simulink model "pid_line_following"  (R2016b)
settings: Solver=FixedStepAuto  StartTime=0.0  StopTime=10.0  RelTol=1e-3  EnableMultiTasking=on
libraries: legoev3lib x6
settings Model: ExtModeTrigDuration=2  Creator=Nexel  LastModifiedBy=Nexel
settings SolverCC: PositivePriorityOrder=on
settings OptimizationCC: MaxStackSize=64
settings DebuggingCC: ParameterTunabilityLossMsg=error
settings HardwareCC: ProdBitPerPointer=32  ProdBitPerSizeT=32  ProdBitPerPtrDiffT=32  ProdLargestAtomicInteger=Long  ProdWordSize=32  ProdHWDeviceType=ARM Compatible->ARM 9
settings RTWCC: SystemTargetFile=ert.tlc  HardwareBoard=LEGO MINDSTORMS EV3  TLCOptions="-aInlineSetEventsForThisBaseRateFcn=TLC_FALSE -aSuppressMultiTaskScheduler=TLC_FALSE  -aRateBasedStepFcn=0"  TemplateMakefile=ert_default_tmf  Description=Embedded Coder  GenerateReport=on  Toolchain=Sourcery G++ Lite v2009q3  IncludeHyperlinkInReport=on  LaunchReport=on  GenerateTraceInfo=on  GenerateTraceReport=on  GenerateTraceReportSl=on  GenerateTraceReportSf=on  GenerateTraceReportEml=on
settings CodeAppCC: ForceParamTrailComments=on  IgnoreCustomStorageClasses=off  OperatorAnnotations=on  SimulinkDataObjDesc=on  SFDataObjDesc=on  MATLABFcnDesc=on  InsertBlockDesc=on  MATLABSourceComments=on
settings ERTTargetCC: SupportContinuousTime=on  SupportVariableSizeSignals=on

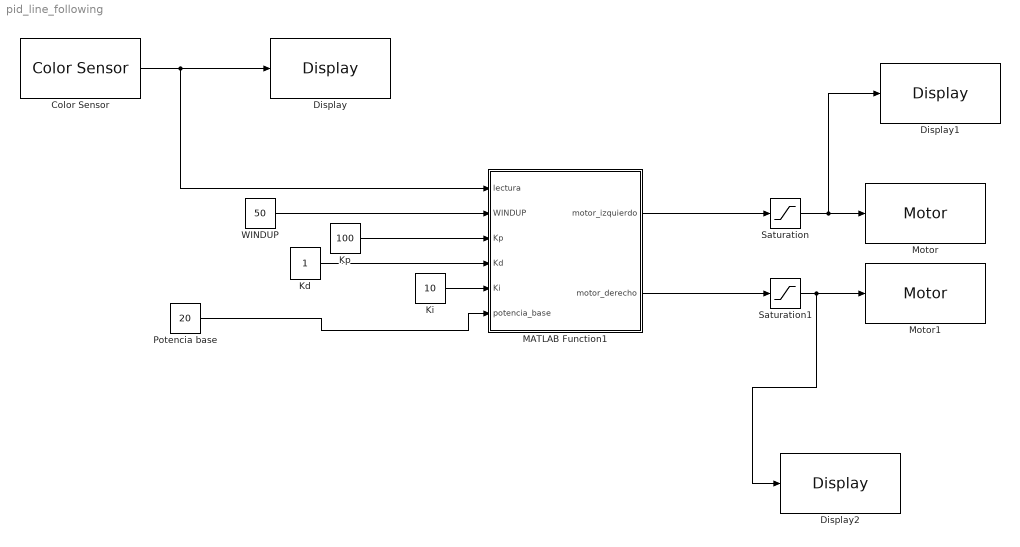
== system pid_line_following ==
  Color Sensor : legoev3lib/Color Sensor  portNumber=1  mode=Reflected light intensity  sampleTime=0.1
  Display : legoev3lib/Display  slcdStr=Gc  slcdLine=2  slcdFormat=Decimal
  Display1 : legoev3lib/Display  slcdStr=Left  slcdLine=3  slcdFormat=Decimal
  Display2 : legoev3lib/Display  slcdStr=Right  slcdLine=4  slcdFormat=Decimal
  Kd : Constant
  Ki : Constant  Value=10
  "Kp " : Constant  Value=100
  MATLAB Function1 : MATLAB Function  TreatAsAtomicUnit=on
  Motor : legoev3lib/Motor  sportNumber=B  sstopAction=Brake
  Motor1 : legoev3lib/Motor  sportNumber=C  sstopAction=Brake
  Potencia base : Constant  Value=20
  Saturation : Saturate  UpperLimit=50  LowerLimit=-50
  Saturation1 : Saturate  UpperLimit=50  LowerLimit=-50
  WINDUP : Constant  Value=50
  wires:
  Color Sensor/1 -> Display/1, MATLAB Function1/1(lectura)
  Potencia base/1 -> MATLAB Function1/6(potencia_base)
  Kd/1 -> MATLAB Function1/4(Kd)
  WINDUP/1 -> MATLAB Function1/2(WINDUP)
  "Kp "/1 -> MATLAB Function1/3(Kp)
  Ki/1 -> MATLAB Function1/5(Ki)
  MATLAB Function1/2(motor_derecho) -> Saturation1/1
  MATLAB Function1/1(motor_izquierdo) -> Saturation/1
  Saturation/1 -> Display1/1, Motor/1
  Saturation1/1 -> Display2/1, Motor1/1

== matlab function pid_line_following/MATLAB Function1 ==
  data: lectura input; WINDUP input; Kp input; Kd input; Ki input; motor_izquierdo output; motor_derecho output; potencia_base input
function [motor_izquierdo, motor_derecho]    = calibrar_luz_sensor(lectura, WINDUP, Kp, Kd, Ki, potencia_base)
    negro = double(5);
    blanco = double(72);
    NEGRO = double(35);
    BLANCO = double(70);
    
    lectura = double(lectura);
    lectura_recta = double((lectura*(BLANCO-NEGRO)/(blanco-negro))+((negro*(BLANCO-NEGRO))+(NEGRO*(blanco-negro)))/(blanco-negro));
    error = lectura_recta-(BLANCO+NEGRO)/2.0;

    persistent s;
    persistent integral;
    persistent previous_error;
    if isempty(s)
        integral = 0;
        s = 1;
        previous_error = 0;
    end
    D = 0.1;
    
    integral = integral + double(error)*D;
    derivada = (error-previous_error) * D;
    previous_error = double(error);
    if abs(integral) > WINDUP
        integral = 0;
    end
        Gc = double(Kp*double(error) + Kd*derivada + Ki*integral);
        Gc = double(Gc/100);
        motor_izquierdo = potencia_base + Gc;
        motor_derecho = potencia_base - Gc;
end
